simulink model "Project1_400100792"  (R2021b)
settings: Solver=VariableStepAuto  StartTime=0.0  StopTime=50  RelTol=1e-3
undefined symbols (not defined in the file or in its folder): eng, gbx, road, tire, veh
settings Model: Creator=baten  LastModifiedBy=baten

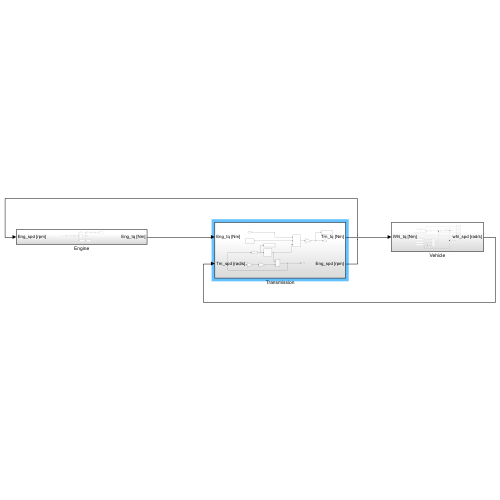
[thumbnail: Simulink's stored preview of the top-level diagram]
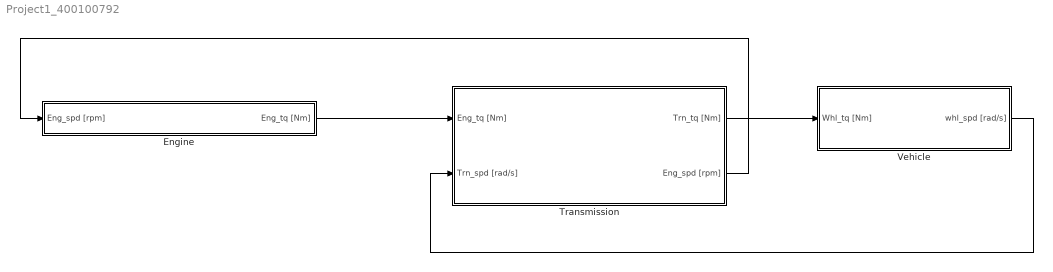
== system Project1_400100792 ==
  Engine : Subsystem
  Transmission : Subsystem
  Vehicle : Subsystem
  wires:
  Engine/1(Eng_tq [Nm]) -> Transmission/1(Eng_tq [Nm])
  Transmission/1(Trn_tq [Nm]) -> Vehicle/1(Whl_tq [Nm])
  Vehicle/1(whl_spd [rad/s]) -> Transmission/2(Trn_spd [rad/s])
  Transmission/2(Eng_spd [rpm]) -> Engine/1(Eng_spd [rpm])

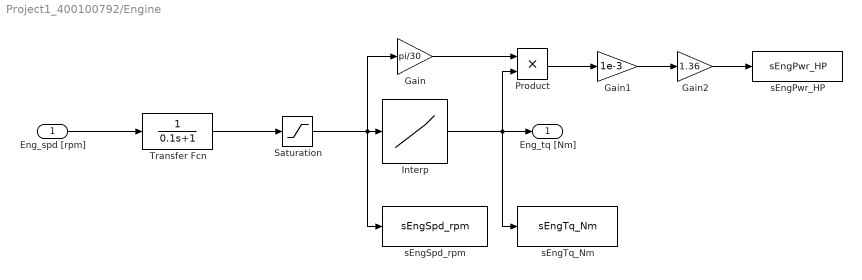
== system Project1_400100792/Engine ==
  Eng_spd [rpm] : Inport
  Gain : Gain  Gain=pi/30
  Gain1 : Gain  Gain=1e-3
  Gain2 : Gain  Gain=1.36
  Interp : Lookup_n-D  NumberOfTableDimensions=1  BreakpointsForDimension1=eng.NtqFullLoad  Table=eng.tqFullLoad  InternalRulePriority=Speed  RndMeth=Simplest  InputSameDT=on
  Product : Product
  Saturation : Saturate  UpperLimit=eng.Nmax  LowerLimit=eng.Nmin
  Transfer Fcn : TransferFcn  Denominator=[0.1 1]
  sEngPwr_HP : ToWorkspace  VariableName=sEngPwr_HP  SampleTime=-1
  sEngSpd_rpm : ToWorkspace  VariableName=sEngSpd_rpm  SampleTime=-1
  sEngTq_Nm : ToWorkspace  VariableName=sEngTq_Nm  SampleTime=-1
  Eng_tq [Nm] : Outport
  wires:
  Gain1/1 -> Gain2/1
  Saturation/1 -> sEngSpd_rpm/1, Gain/1, Interp/1
  Interp/1 -> Eng_tq [Nm]/1, sEngTq_Nm/1, Product/2
  Transfer Fcn/1 -> Saturation/1
  Product/1 -> Gain1/1
  Eng_spd [rpm]/1 -> Transfer Fcn/1
  Gain/1 -> Product/1
  Gain2/1 -> sEngPwr_HP/1

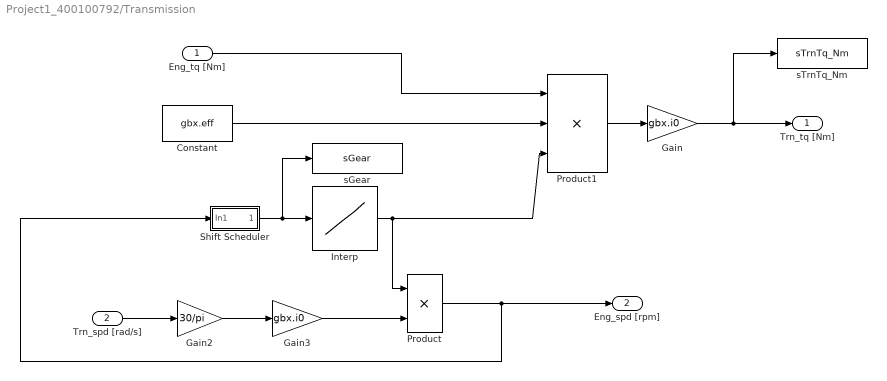
== system Project1_400100792/Transmission ==
  Eng_tq [Nm] : Inport
  Trn_spd [rad/s] : Inport  Port=2
  Constant : Constant  Value=gbx.eff
  Gain : Gain  Gain=gbx.i0
  Gain2 : Gain  Gain=30/pi
  Gain3 : Gain  Gain=gbx.i0
  Interp : Lookup_n-D  NumberOfTableDimensions=1  BreakpointsForDimension1=[1:8]  Table=gbx.gearRat  InternalRulePriority=Speed  RndMeth=Simplest  InputSameDT=on
  Product : Product
  Product1 : Product  Inputs=3
  Shift Scheduler : Subsystem
  sGear : ToWorkspace  VariableName=sGear  SampleTime=-1
  sTrnTq_Nm : ToWorkspace  VariableName=sTrnTq_Nm  SampleTime=-1
  Trn_tq [Nm] : Outport
  Eng_spd [rpm] : Outport  Port=2
  wires:
  Eng_tq [Nm]/1 -> Product1/1
  Trn_spd [rad/s]/1 -> Gain2/1
  Shift Scheduler/1(Out1) -> sGear/1, Interp/1
  Interp/1 -> Product1/3, Product/1
  Product/1 -> Eng_spd [rpm]/1, Shift Scheduler/1(In1)
  Gain2/1 -> Gain3/1
  Gain3/1 -> Product/2
  Product1/1 -> Gain/1
  Gain/1 -> sTrnTq_Nm/1, Trn_tq [Nm]/1
  Constant/1 -> Product1/2

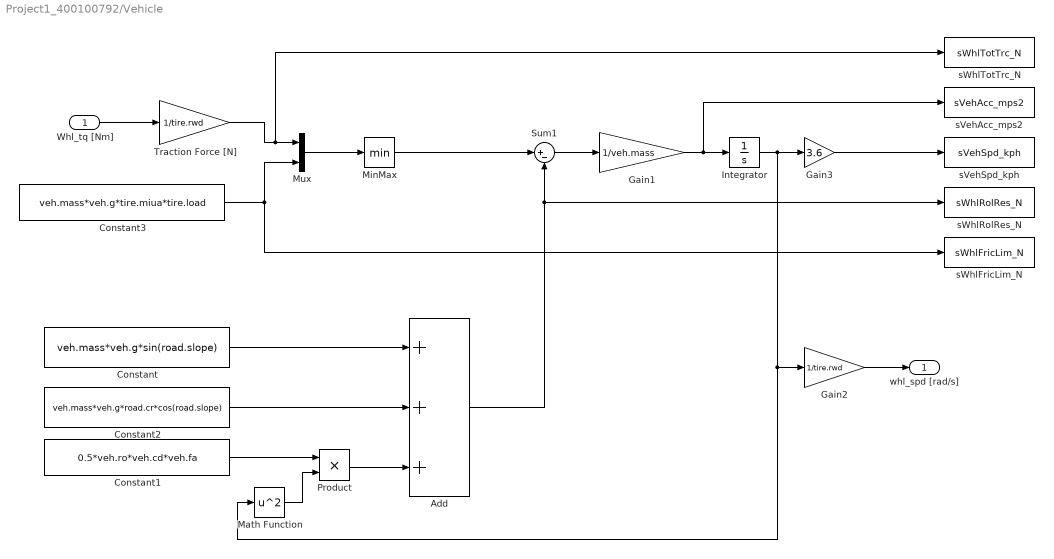
== system Project1_400100792/Vehicle ==
  Whl_tq [Nm] : Inport
  Add : Sum  Inputs=+++
  Constant : Constant  Value=veh.mass*veh.g*sin(road.slope)
  Constant1 : Constant  Value=0.5*veh.ro*veh.cd*veh.fa
  Constant2 : Constant  Value=veh.mass*veh.g*road.cr*cos(road.slope)
  Constant3 : Constant  Value=veh.mass*veh.g*tire.miua*tire.load
  Gain1 : Gain  Gain=1/veh.mass
  Gain2 : Gain  Gain=1/tire.rwd
  Gain3 : Gain  Gain=3.6
  Integrator : Integrator  LimitOutput=on  LowerSaturationLimit=0
  Math Function : Math  Operator=square  SaturateOnIntegerOverflow=on
  MinMax : MinMax
  Mux : Mux  Inputs=2
  Product : Product
  Sum1 : Sum  Inputs=|+-
  Traction Force [N] : Gain  Gain=1/tire.rwd
  sVehAcc_mps2 : ToWorkspace  VariableName=sVehAcc_mps2  SampleTime=-1
  sVehSpd_kph : ToWorkspace  VariableName=sVehSpd_kph  SampleTime=-1
  sWhlFricLim_N : ToWorkspace  VariableName=sWhlFricLim_N  SampleTime=-1
  sWhlRolRes_N : ToWorkspace  VariableName=sWhlRolRes_N  SampleTime=-1
  sWhlTotTrc_N : ToWorkspace  VariableName=sWhlTotTrc_N  SampleTime=-1
  whl_spd [rad/s] : Outport
  wires:
  Constant3/1 -> Mux/2, sWhlFricLim_N/1
  Mux/1 -> MinMax/1
  Constant2/1 -> Add/2
  Constant/1 -> Add/1
  Gain3/1 -> sVehSpd_kph/1
  Integrator/1 -> Gain2/1, Math Function/1, Gain3/1
  Add/1 -> sWhlRolRes_N/1, Sum1/2
  Traction Force [N]/1 -> sWhlTotTrc_N/1, Mux/1
  Math Function/1 -> Product/2
  Gain1/1 -> Integrator/1, sVehAcc_mps2/1
  Gain2/1 -> whl_spd [rad/s]/1
  Whl_tq [Nm]/1 -> Traction Force [N]/1
  Sum1/1 -> Gain1/1
  Constant1/1 -> Product/1
  Product/1 -> Add/3
  MinMax/1 -> Sum1/1

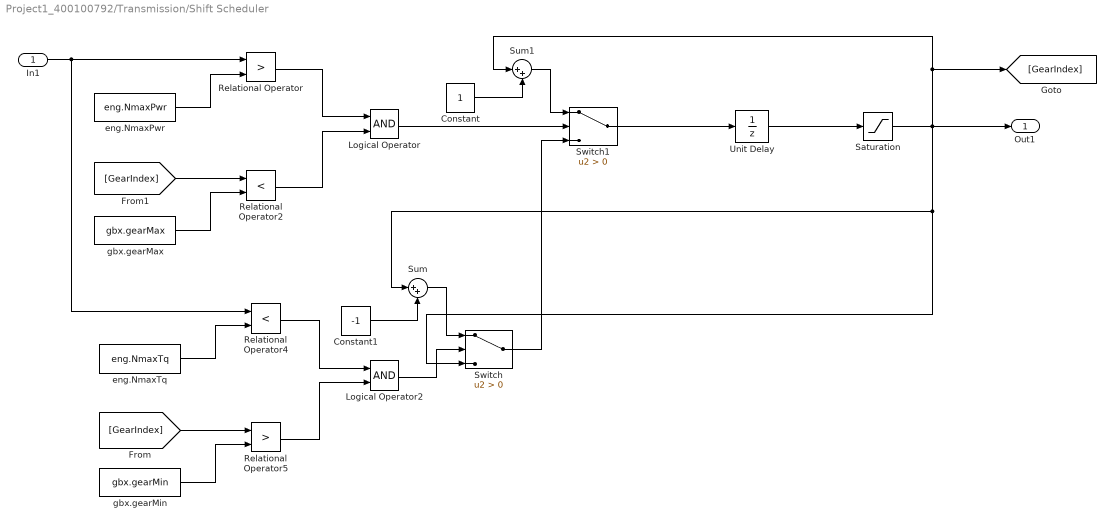
== system Project1_400100792/Transmission/Shift Scheduler ==
  In1 : Inport
  Constant : Constant
  Constant1 : Constant  Value=-1
  Logical Operator : Logic  AllPortsSameDT=off  OutDataTypeStr=boolean
  Logical Operator2 : Logic  AllPortsSameDT=off  OutDataTypeStr=boolean
  Relational Operator : RelationalOperator  Operator=>  OutDataTypeStr=boolean  RndMeth=Simplest
  Relational Operator2 : RelationalOperator  Operator=<  OutDataTypeStr=boolean  RndMeth=Simplest
  Relational Operator4 : RelationalOperator  Operator=<  OutDataTypeStr=boolean  RndMeth=Simplest
  Relational Operator5 : RelationalOperator  Operator=>  OutDataTypeStr=boolean  RndMeth=Simplest
  Saturation : Saturate  UpperLimit=8  LowerLimit=1
  Sum : Sum  Inputs=|++
  Sum1 : Sum  Inputs=|++
  Switch : Switch  Criteria=u2 > Threshold
  Switch1 : Switch  Criteria=u2 > Threshold
  Unit Delay : UnitDelay  SampleTime=-1  HasFrameUpgradeWarning=on
  eng.NmaxPwr : Constant  Value=eng.NmaxPwr
  eng.NmaxTq : Constant  Value=eng.NmaxTq
  gbx.gearMax : Constant  Value=gbx.gearMax
  gbx.gearMin : Constant  Value=gbx.gearMin
  Out1 : Outport
  wires:
  In1/1 -> Relational Operator4/1, Relational Operator/1
  eng.NmaxPwr/1 -> Relational Operator/2
  gbx.gearMax/1 -> Relational Operator2/2
  Relational Operator/1 -> Logical Operator/1
  Relational Operator2/1 -> Logical Operator/2
  gbx.gearMin/1 -> Relational Operator5/2
  eng.NmaxTq/1 -> Relational Operator4/2
  Relational Operator5/1 -> Logical Operator2/2
  Relational Operator4/1 -> Logical Operator2/1
  Logical Operator/1 -> Switch1/2
  Sum1/1 -> Switch1/1
  Logical Operator2/1 -> Switch/2
  Sum/1 -> Switch/1
  Constant/1 -> Sum1/2
  Constant1/1 -> Sum/2
  Switch1/1 -> Unit Delay/1
  Unit Delay/1 -> Saturation/1
  Saturation/1 -> Switch/3, Sum/1, [GearIndex], Sum1/1, Out1/1
  Switch/1 -> Switch1/3
  [GearIndex] -> Relational Operator5/1
  [GearIndex] -> Relational Operator2/1
